simulink model "mehrw3"  (Simulink 4.00)
settings: Solver=ode45  SolverMode=SingleTasking  StartTime=0.0  StopTime=30  FixedStep=0.1  MaxStep=0.1  RelTol=1e-3  AbsTol=1e-6
values from neighbouring files (symbols this model uses):
  A = zeros(10,10);			A(1:5,6:10) = eye(5,5)    [mehrw_1.m]    (also in mehrw_2.m; mehrw_3.m; mehrw_4.m; mehrw_5.m)
  B = [zeros(5,2); 1, 0; zeros(3,2); 0, -1]    [mehrw_1.m]    (also in mehrw_2.m; mehrw_3.m; mehrw_4.m; mehrw_5.m)
  C = 500e-6    (= 0.0005)    [inv_switch_1.m]    (also in mehrw_1.m = eye(10,10); mehrw_2.m = eye(10,10); mehrw_3.m = eye(10,10); mehrw_4.m = eye(10,10))
  Cy = zeros(1,10);				Cy(1,10) = 1    [mehrw_1.m]    (also in mehrw_2.m; mehrw_3.m; mehrw_4.m; mehrw_5.m)
  D = 100    [behaelter_1.m]    (also in behaelter_2.m; mehrw_1.m = zeros(10,2); mehrw_2.m = zeros(10,2); mehrw_3.m = zeros(10,2))
  rT = 0.1    [mehrw_1.m]    (also in mehrw_2.m; mehrw_3.m; mehrw_4.m; mehrw_5.m)
settings Model: LastModifiedBy=Administrator  Refine=3  SaveTime=off  SaveOutput=off  LimitDataPoints=off  BlockReductionOpt=off

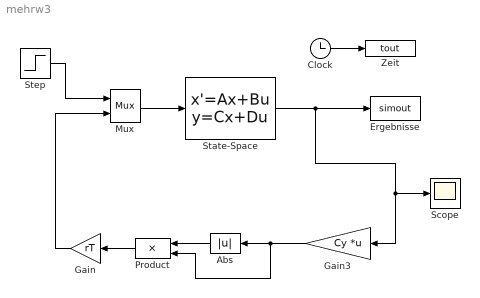
== system mehrw3 ==
  Abs : Abs  Orientation=left  SaturateOnIntegerOverflow=on
  Clock : Clock
      settings: DisplayTime=off  Decimation=10
  Ergebnisse : ToWorkspace  VariableName=simout  SampleTime=0  SaveFormat=Array
      settings: MaxDataPoints=1000
  Gain : Gain  Orientation=left  Gain=rT  Multiplication=Element-wise(K.*u)  SaturateOnIntegerOverflow=on
  Gain3 : Gain  Orientation=left  Gain=Cy  Multiplication=Matrix(K*u)  SaturateOnIntegerOverflow=on
  Mux : Mux  Inputs=2
      settings: DisplayOption=none
  Product : Product  Orientation=left  Inputs=2  Multiplication=Element-wise(.*)  SaturateOnIntegerOverflow=on
  Scope : Scope
      settings: TickLabels=on  TimeRange=30  YMin=-41.6038  YMax=41.6038  SaveToWorkspace=off  SaveName=ScopeData  DataFormat=Array  LimitDataPoints=on  MaxDataPoints=5000
  State-Space : StateSpace  A=A  B=B  C=C  D=D  X0=0  Realization=auto  AbsoluteTolerance=auto
  Step : Step  Time=0  Before=0  After=1  SampleTime=0
  Zeit : ToWorkspace  VariableName=tout  SampleTime=0  SaveFormat=Array
      settings: MaxDataPoints=1000
  wires:
  Gain3/1 -> Product/2, Abs/1
  Product/1 -> Gain/1
  Gain/1 -> Mux/2
  Abs/1 -> Product/1
  Step/1 -> Mux/1
  Mux/1 -> State-Space/1
  Clock/1 -> Zeit/1
  State-Space/1 -> Ergebnisse/1, Gain3/1, Scope/1
